simulink model "plantModel_cart_signalFlow"  (R2023b)
settings: Solver=ode4  StartTime=0.0  StopTime=10.0  FixedStep=1e-2  RelTol=1e-3
settings Model: Creator=evreng  LastModifiedBy=evreng

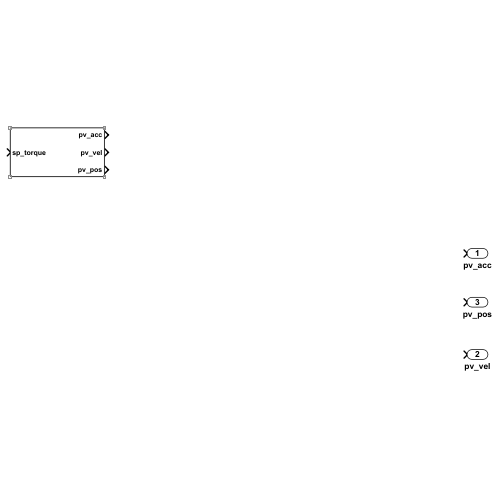
[thumbnail: Simulink's stored preview of the top-level diagram]
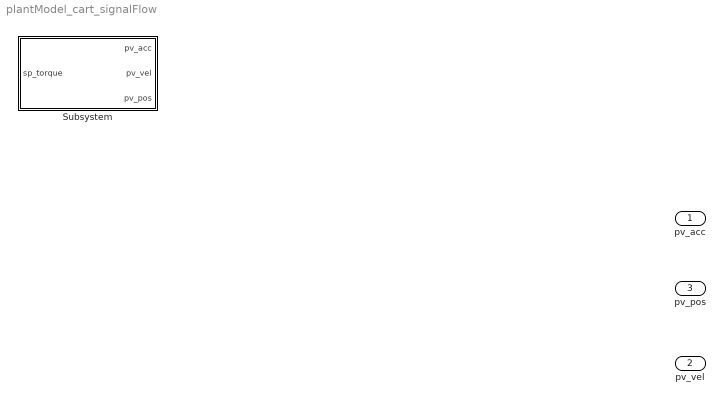
== system plantModel_cart_signalFlow ==
  Subsystem : Subsystem
  pv_acc : Outport
  pv_vel : Outport  Port=2
  pv_pos : Outport  Port=3

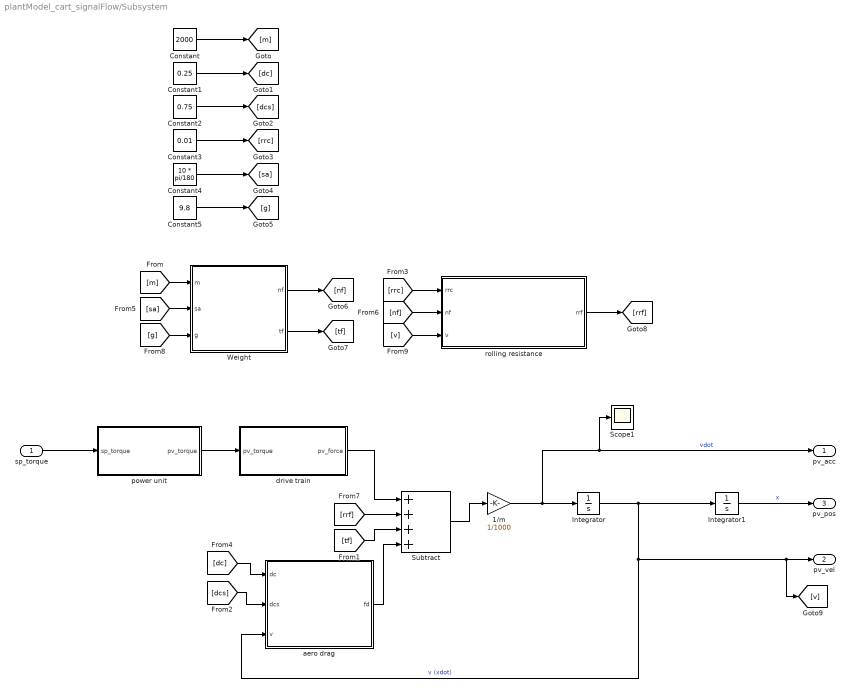
== system plantModel_cart_signalFlow/Subsystem ==
  sp_torque : Inport
  1/m : Gain  Gain=1/1000
  Constant : Constant  Value=2000
  Constant1 : Constant  Value=0.25
  Constant2 : Constant  Value=0.75
  Constant3 : Constant  Value=0.01
  Constant4 : Constant  Value=10 * pi/180
  Constant5 : Constant  Value=9.8
  Integrator : Integrator
  Integrator1 : Integrator
  Scope1 : Scope
  Subtract : Sum  Inputs=++++
  Weight : MATLAB Function  TreatAsAtomicUnit=on
  aero drag : MATLAB Function  TreatAsAtomicUnit=on
  drive train : Subsystem
  power unit : Subsystem
  rolling resistance : MATLAB Function  TreatAsAtomicUnit=on
  pv_acc : Outport
  pv_vel : Outport  Port=2
  pv_pos : Outport  Port=3
  wires:
  [v] -> rolling resistance/3(v)
  [m] -> Weight/1(m)
  Constant/1 -> [m]
  sp_torque/1 -> power unit/1(sp_torque)
  [g] -> Weight/3(g)
  Constant3/1 -> [rrc]
  [dc] -> aero drag/1(dc)
  [tf] -> Subtract/3
  1/m/1 -> Integrator/1, pv_acc/1, Scope1/1  "vdot"
  [nf] -> rolling resistance/2(nf)
  [sa] -> Weight/2(sa)
  Weight/1(nf) -> [nf]
  Constant2/1 -> [dcs]
  Weight/2(tf) -> [tf]
  Integrator1/1 -> pv_pos/1  "x"
  drive train/1(pv_force) -> Subtract/1
  Constant5/1 -> [g]
  rolling resistance/1(rrf) -> [rrf]
  aero drag/1(fd) -> Subtract/4
  Subtract/1 -> 1/m/1
  Constant1/1 -> [dc]
  Constant4/1 -> [sa]
  [rrc] -> rolling resistance/1(rrc)
  Integrator/1 -> aero drag/3(v), pv_vel/1, [v], Integrator1/1  "v (xdot)"
  [dcs] -> aero drag/2(dcs)
  [rrf] -> Subtract/2
  power unit/1(pv_torque) -> drive train/1(pv_torque)

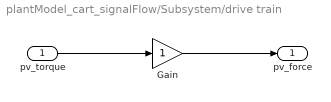
== system plantModel_cart_signalFlow/Subsystem/drive train ==
  pv_torque : Inport
  Gain : Gain
  pv_force : Outport
  wires:
  pv_torque/1 -> Gain/1
  Gain/1 -> pv_force/1

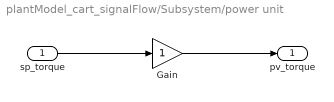
== system plantModel_cart_signalFlow/Subsystem/power unit ==
  sp_torque : Inport
  Gain : Gain
  pv_torque : Outport
  wires:
  sp_torque/1 -> Gain/1
  Gain/1 -> pv_torque/1

== matlab function plantModel_cart_signalFlow/Subsystem/rolling resistance ==
  data: rrc input; rrf output; nf input; v input
function rrf = rollingResistance(rrc, nf, v)
tol = 1e-3;
if abs(v) > tol
    rrf = rrc * nf * (-1 * sign(v));
else
    rrf = 0;
end

== matlab function plantModel_cart_signalFlow/Subsystem/aero drag ==
  data: dc input; fd output; dcs input; v input
function fd = aeroDrag(dc, dcs, v)
fd = 0.5 * dc * dcs * v ^ 2 * (-1 * sign(v));

== matlab function plantModel_cart_signalFlow/Subsystem/Weight ==
  data: m input; nf output; sa input; tf output; g input
function [nf, tf] = fcn(m, sa, g)
nf = m * g * cos(sa);
tf = -1 * m * g * sin(sa);
